simulink library "halin"  (R2021b)
settings: Solver=VariableStepAuto  StartTime=0.0  StopTime=10.0  RelTol=1e-3
undefined symbols (not defined in the file): KHAL_CAN1ABM1E2E_flg, KHAL_CAN1ESC1E2E_flg, KHAL_CAN1ESC5E2E_flg, KHAL_CAN1ESC7E2E_flg, KHAL_CAN1FCM2E2E_flg, KHAL_CAN1FCM3E2E_flg, KHAL_CAN1FCM4E2E_flg, KHAL_CAN3BMS1E2E_flg, KHAL_CAN3BMS6E2E_flg, KHAL_CAN3CCU1E2E_flg, KHAL_CAN3CCU2E2E_flg, KHAL_CAN3MCUF1E2E_flg, KHAL_CAN3MCUR1E2E_flg, KHAL_CAN3Shifter1E2E_flg, TRUE
libraries: simulink x420, FVT_lib x149, hcu_lib x49
(part 1 of 14)
settings Model: Creator=13168  LastModifiedBy=FVT23118
settings SolverCC: AlgebraicLoopSolver=TrustRegion
settings DataIOCC: SaveFormat=Array  SignalLoggingSaveFormat=ModelDataLogs  ReturnWorkspaceOutputs=off
settings OptimizationCC: BlockReduction=off  BooleanDataType=off
settings DebuggingCC: SaveWithParameterizedLinksMsg=none  UnderspecifiedInitializationDetection=Classic  MergeDetectMultiDrivingBlocksExec=none  SignalResolutionControl=TryResolveAllWithWarning  SFMachineParentedDataDiag=warning
settings HardwareCC: TargetUnknown=on
settings ModelReferenceCC: PropagateSignalLabelsOutOfModel=off
settings ConfigComp: CovMetricSettings=dw  CovSaveCumulativeToWorkspaceVar=on  CovSaveSingleToWorkspaceVar=on

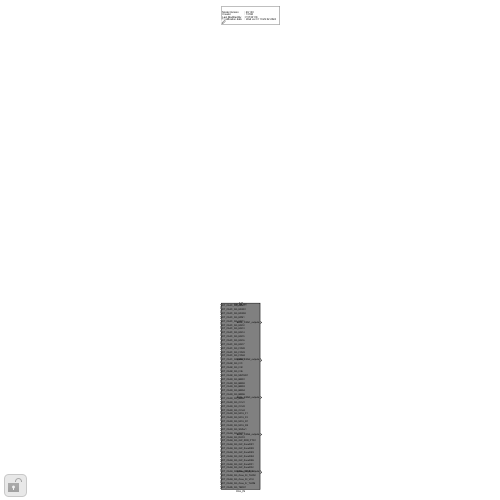
[thumbnail: Simulink's stored preview of the top-level diagram]
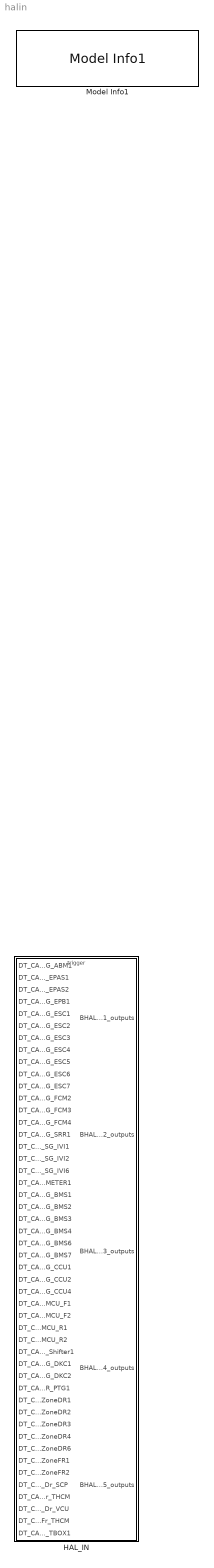
== system halin ==
  HAL_IN : Subsystem
      settings: RTWSystemCode=Nonreusable function  RTWFcnNameOpts=Use subsystem name  RTWFileNameOpts=Use subsystem name
  Model Info1 : hcu_lib/Model Info1  BlockCM=None  Frame=on  DisplayStringWithTags=|  HorizontalTextAlignment=Left  LeftAlignmentValue=0.02  SourceBlockDiagram=hcu_lib  TagMaxNumber=20
      | Model Version        : %<ModelVersion>
      | Creator                   : %<Creator>
      | Last Modified By    : %<LastModifiedBy>
      | Modification date    : %<LastModificationDate>
      settings: SourceProductName=HCU Relative Block Library

== system halin/HAL_IN ==
  DT_CAN1_SG_ABM1 : Inport
  DT_CAN1_SG_EPAS1 : Inport  Port=2
  DT_CAN1_SG_EPAS2 : Inport  Port=3
  DT_CAN1_SG_EPB1 : Inport  Port=4
  DT_CAN1_SG_ESC1 : Inport  Port=5
  DT_CAN1_SG_ESC2 : Inport  Port=6
  DT_CAN1_SG_ESC3 : Inport  Port=7
  DT_CAN1_SG_ESC4 : Inport  Port=8
  DT_CAN1_SG_ESC5 : Inport  Port=9
  DT_CAN1_SG_ESC6 : Inport  Port=10
  DT_CAN1_SG_ESC7 : Inport  Port=11
  DT_CAN1_SG_FCM2 : Inport  Port=12
  DT_CAN1_SG_FCM3 : Inport  Port=13
  DT_CAN1_SG_FCM4 : Inport  Port=14
  DT_CAN1_SG_SRR1 : Inport  Port=15
  DT_CAN2_SG_IVI1 : Inport  Port=16
  DT_CAN2_SG_IVI2 : Inport  Port=17
  DT_CAN2_SG_IVI6 : Inport  Port=18
  DT_CAN2_SG_METER1 : Inport  Port=19
  DT_CAN3_SG_BMS1 : Inport  Port=20
  DT_CAN3_SG_BMS2 : Inport  Port=21
  DT_CAN3_SG_BMS3 : Inport  Port=22
  DT_CAN3_SG_BMS4 : Inport  Port=23
  DT_CAN3_SG_BMS6 : Inport  Port=24
  DT_CAN3_SG_BMS7 : Inport  Port=25
  DT_CAN3_SG_CCU1 : Inport  Port=26
  DT_CAN3_SG_CCU2 : Inport  Port=27
  DT_CAN3_SG_CCU4 : Inport  Port=28
  DT_CAN3_SG_MCU_F1 : Inport  Port=29
  DT_CAN3_SG_MCU_F2 : Inport  Port=30
  DT_CAN3_SG_MCU_R1 : Inport  Port=31
  DT_CAN3_SG_MCU_R2 : Inport  Port=32
  DT_CAN3_SG_Shifter1 : Inport  Port=33
  DT_CAN4_SG_DKC1 : Inport  Port=34
  DT_CAN4_SG_DKC2 : Inport  Port=35
  DT_CAN4_SG_GW_ZDR_PTG1 : Inport  Port=36
  DT_CAN4_SG_GW_ZoneDR1 : Inport  Port=37
  DT_CAN4_SG_GW_ZoneDR2 : Inport  Port=38
  DT_CAN4_SG_GW_ZoneDR3 : Inport  Port=39
  DT_CAN4_SG_GW_ZoneDR4 : Inport  Port=40
  DT_CAN4_SG_GW_ZoneDR6 : Inport  Port=41
  DT_CAN4_SG_GW_ZoneFR1 : Inport  Port=42
  DT_CAN4_SG_GW_ZoneFR2 : Inport  Port=43
  DT_CAN4_SG_Zone_Dr_SCP : Inport  Port=44
  DT_CAN4_SG_Zone_Dr_THCM : Inport  Port=45
  DT_CAN4_SG_Zone_Dr_VCU : Inport  Port=46
  DT_CAN4_SG_Zone_Fr_THCM : Inport  Port=47
  DT_CAN5_SG_TBOX1 : Inport  Port=48
  trig_hal_in : TriggerPort  TriggerType=function-call  VariantControl=(inherit)
  CAN1 : Subsystem
  CAN2 : Subsystem
  CAN3 : Subsystem
  CAN4 : Subsystem
  CAN5 : Subsystem
  BHAL_CAN1_outputs : Outport  OutDataTypeStr=Bus: BHAL_CAN1_outputs
  BHAL_CAN2_outputs : Outport  Port=2  OutDataTypeStr=Bus: BHAL_CAN2_outputs
  BHAL_CAN3_outputs : Outport  Port=3  OutDataTypeStr=Bus: BHAL_CAN3_outputs
  BHAL_CAN4_outputs : Outport  Port=4  OutDataTypeStr=Bus: BHAL_CAN4_outputs
  BHAL_CAN5_outputs : Outport  Port=5  OutDataTypeStr=Bus: BHAL_CAN5_outputs
  wires:
  DT_CAN3_SG_CCU1/1 -> CAN3/7(DT_CAN3_SG_CCU1)
  DT_CAN3_SG_BMS3/1 -> CAN3/3(DT_CAN3_SG_BMS3)
  DT_CAN3_SG_BMS4/1 -> CAN3/4(DT_CAN3_SG_BMS4)
  DT_CAN3_SG_BMS2/1 -> CAN3/2(DT_CAN3_SG_BMS2)
  DT_CAN3_SG_MCU_R2/1 -> CAN3/13(DT_CAN3_SG_MCU_R2)
  DT_CAN3_SG_MCU_R1/1 -> CAN3/12(DT_CAN3_SG_MCU_R1)
  DT_CAN3_SG_BMS6/1 -> CAN3/5(DT_CAN3_SG_BMS6)
  DT_CAN3_SG_MCU_F1/1 -> CAN3/10(DT_CAN3_SG_MCU_F1)
  DT_CAN3_SG_MCU_F2/1 -> CAN3/11(DT_CAN3_SG_MCU_F2)
  DT_CAN3_SG_BMS1/1 -> CAN3/1(DT_CAN3_SG_BMS1)
  DT_CAN3_SG_CCU2/1 -> CAN3/8(DT_CAN3_SG_CCU2)
  DT_CAN4_SG_DKC2/1 -> CAN4/2(DT_CAN4_SG_DKC2)
  DT_CAN4_SG_DKC1/1 -> CAN4/1(DT_CAN4_SG_DKC1)
  DT_CAN4_SG_GW_ZDR_PTG1/1 -> CAN4/3(DT_CAN4_SG_GW_ZDR_PTG1)
  DT_CAN3_SG_CCU4/1 -> CAN3/9(DT_CAN3_SG_CCU4)
  DT_CAN4_SG_Zone_Dr_VCU/1 -> CAN4/13(DT_CAN4_SG_Zone_Dr_VCU)
  DT_CAN4_SG_Zone_Dr_SCP/1 -> CAN4/11(DT_CAN4_SG_Zone_Dr_SCP)
  DT_CAN4_SG_Zone_Dr_THCM/1 -> CAN4/12(DT_CAN4_SG_Zone_Dr_THCM)
  DT_CAN4_SG_GW_ZoneDR3/1 -> CAN4/6(DT_CAN4_SG_GW_ZoneDR3)
  CAN3/1(HAL_CAN3_outputs) -> BHAL_CAN3_outputs/1
  DT_CAN4_SG_GW_ZoneDR6/1 -> CAN4/8(DT_CAN4_SG_GW_ZoneDR6)
  CAN2/1(HAL_CAN2_outputs) -> BHAL_CAN2_outputs/1
  DT_CAN2_SG_METER1/1 -> CAN2/4(DT_CAN2_SG_METER1)
  DT_CAN4_SG_GW_ZoneFR1/1 -> CAN4/9(DT_CAN4_SG_GW_ZoneFR1)
  DT_CAN2_SG_IVI2/1 -> CAN2/2(DT_CAN2_SG_IVI2)
  DT_CAN2_SG_IVI1/1 -> CAN2/1(DT_CAN2_SG_IVI1)
  DT_CAN2_SG_IVI6/1 -> CAN2/3(DT_CAN2_SG_IVI6)
  DT_CAN1_SG_FCM3/1 -> CAN1/13(DT_CAN1_SG_FCM3)
  DT_CAN1_SG_FCM2/1 -> CAN1/12(DT_CAN1_SG_FCM2)
  DT_CAN1_SG_ESC7/1 -> CAN1/11(DT_CAN1_SG_ESC7)
  DT_CAN4_SG_GW_ZoneDR1/1 -> CAN4/4(DT_CAN4_SG_GW_ZoneDR1)
  DT_CAN1_SG_ESC6/1 -> CAN1/10(DT_CAN1_SG_ESC6)
  DT_CAN4_SG_GW_ZoneDR4/1 -> CAN4/7(DT_CAN4_SG_GW_ZoneDR4)
  DT_CAN3_SG_Shifter1/1 -> CAN3/14(DT_CAN3_SG_Shifter1)
  DT_CAN1_SG_ESC5/1 -> CAN1/9(DT_CAN1_SG_ESC5)
  DT_CAN4_SG_GW_ZoneFR2/1 -> CAN4/10(DT_CAN4_SG_GW_ZoneFR2)
  DT_CAN1_SG_ESC2/1 -> CAN1/6(DT_CAN1_SG_ESC2)
  DT_CAN1_SG_ESC3/1 -> CAN1/7(DT_CAN1_SG_ESC3)
  DT_CAN1_SG_ESC4/1 -> CAN1/8(DT_CAN1_SG_ESC4)
  DT_CAN1_SG_ESC1/1 -> CAN1/5(DT_CAN1_SG_ESC1)
  DT_CAN1_SG_EPAS2/1 -> CAN1/3(DT_CAN1_SG_EPAS2)
  DT_CAN4_SG_Zone_Fr_THCM/1 -> CAN4/14(DT_CAN4_SG_Zone_Fr_THCM)
  DT_CAN4_SG_GW_ZoneDR2/1 -> CAN4/5(DT_CAN4_SG_GW_ZoneDR2)
  DT_CAN1_SG_EPAS1/1 -> CAN1/2(DT_CAN1_SG_EPAS1)
  DT_CAN1_SG_EPB1/1 -> CAN1/4(DT_CAN1_SG_EPB1)
  CAN4/1(HAL_CAN4_outputs) -> BHAL_CAN4_outputs/1
  DT_CAN1_SG_SRR1/1 -> CAN1/15(DT_CAN1_SG_SRR1)
  DT_CAN1_SG_FCM4/1 -> CAN1/14(DT_CAN1_SG_FCM4)
  DT_CAN1_SG_ABM1/1 -> CAN1/1(DT_CAN1_SG_ABM1)
  DT_CAN5_SG_TBOX1/1 -> CAN5/1(DT_CAN5_SG_TBOX1)
  CAN1/1(HAL_CAN1_outputs) -> BHAL_CAN1_outputs/1
  CAN5/1(HAL_CAN5_outputs) -> BHAL_CAN5_outputs/1
  DT_CAN3_SG_BMS7/1 -> CAN3/6(DT_CAN3_SG_BMS7)

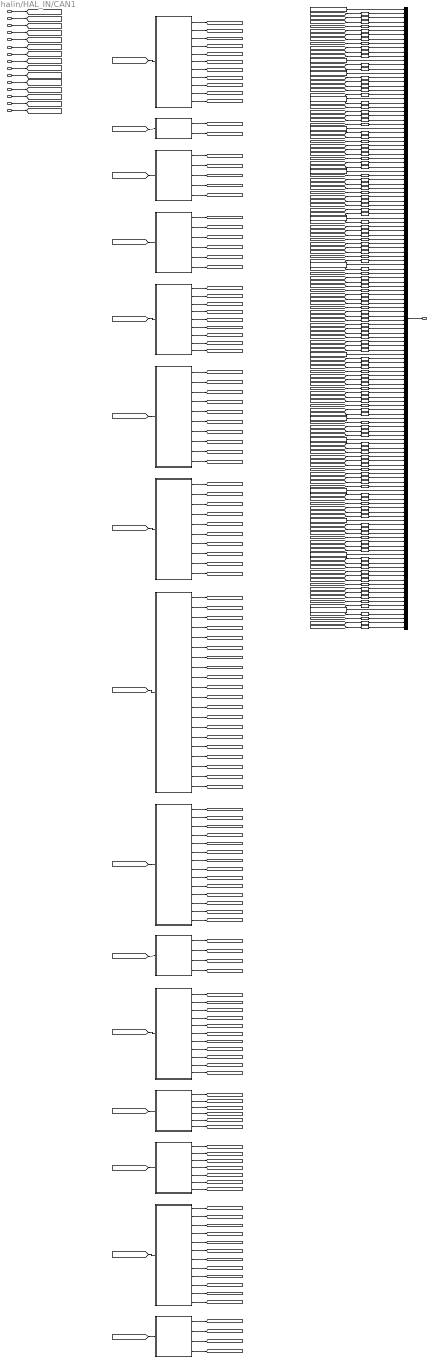
== system halin/HAL_IN/CAN1 ==
  DT_CAN1_SG_ABM1 : Inport
  DT_CAN1_SG_EPAS1 : Inport  Port=2
  DT_CAN1_SG_EPAS2 : Inport  Port=3
  DT_CAN1_SG_EPB1 : Inport  Port=4
  DT_CAN1_SG_ESC1 : Inport  Port=5
  DT_CAN1_SG_ESC2 : Inport  Port=6
  DT_CAN1_SG_ESC3 : Inport  Port=7
  DT_CAN1_SG_ESC4 : Inport  Port=8
  DT_CAN1_SG_ESC5 : Inport  Port=9
  DT_CAN1_SG_ESC6 : Inport  Port=10
  DT_CAN1_SG_ESC7 : Inport  Port=11
  DT_CAN1_SG_FCM2 : Inport  Port=12
  DT_CAN1_SG_FCM3 : Inport  Port=13
  DT_CAN1_SG_FCM4 : Inport  Port=14
  DT_CAN1_SG_SRR1 : Inport  Port=15
  ABM1 : Subsystem
  EPAS1 : Subsystem
  EPAS2 : Subsystem
  EPB1 : Subsystem
  ESC1 : Subsystem
  ESC2 : Subsystem
  ESC3 : Subsystem
  ESC4 : Subsystem
  ESC5 : Subsystem
  ESC6 : Subsystem
  ESC7 : Subsystem
  FCM2 : Subsystem
  FCM3 : Subsystem
  FCM4 : Subsystem
  SRR1 : Subsystem
  UnitConverter{,1..2,5,7..10,14,16..19,21..22,24..25,28,31,34,36,39,41,44,46,49,51,53..62,64..76,80,82,84,86..87,90..92,94,97,101..103,105,108..109,112,115..116,122..124} (72 alike) : DataTypeConversion  OutDataTypeStr=boolean
  UnitConverter{13,15,29..30,32,35,40,45,50,63,79,81,83,85,93,98,100,104,110..111} (20 alike) : DataTypeConversion  OutDataTypeStr=single
  UnitConverter{3..4,6,11..12,20,23,26..27,33,37..38,42..43,47..48,52,77..78,88..89,95..96,99,106..107,113..114,117..121,125..130} (39 alike) : DataTypeConversion  OutDataTypeStr=uint8
  VHAL_CANMsgInvalidABM1_flg : Subsystem  AncestorBlock=FVT_lib/hal/MsgTimeoutJudge_CAN_AUTOSAR
      mask help: MeasumentTrigerEvent
      mask Display: fprintf('MsgTimeoutJudge_CAN\nAUTOSAR');
  VHAL_CANMsgInvalidEPAS1_flg : Subsystem  AncestorBlock=FVT_lib/hal/MsgTimeoutJudge_CAN_AUTOSAR
      mask help: MeasumentTrigerEvent
      mask Display: fprintf('MsgTimeoutJudge_CAN\nAUTOSAR');
  VHAL_CANMsgInvalidEPAS2_flg : Subsystem  AncestorBlock=FVT_lib/hal/MsgTimeoutJudge_CAN_AUTOSAR
      mask help: MeasumentTrigerEvent
      mask Display: fprintf('MsgTimeoutJudge_CAN\nAUTOSAR');
  VHAL_CANMsgInvalidEPB1_flg : Subsystem  AncestorBlock=FVT_lib/hal/MsgTimeoutJudge_CAN_AUTOSAR
      mask help: MeasumentTrigerEvent
      mask Display: fprintf('MsgTimeoutJudge_CAN\nAUTOSAR');
  VHAL_CANMsgInvalidESC1_flg : Subsystem  AncestorBlock=FVT_lib/hal/MsgTimeoutJudge_CAN_AUTOSAR
      mask help: MeasumentTrigerEvent
      mask Display: fprintf('MsgTimeoutJudge_CAN\nAUTOSAR');
  VHAL_CANMsgInvalidESC2_flg : Subsystem  AncestorBlock=FVT_lib/hal/MsgTimeoutJudge_CAN_AUTOSAR
      mask help: MeasumentTrigerEvent
      mask Display: fprintf('MsgTimeoutJudge_CAN\nAUTOSAR');
  VHAL_CANMsgInvalidESC3_flg : Subsystem  AncestorBlock=FVT_lib/hal/MsgTimeoutJudge_CAN_AUTOSAR
      mask help: MeasumentTrigerEvent
      mask Display: fprintf('MsgTimeoutJudge_CAN\nAUTOSAR');
  VHAL_CANMsgInvalidESC4_flg : Subsystem  AncestorBlock=FVT_lib/hal/MsgTimeoutJudge_CAN_AUTOSAR
      mask help: MeasumentTrigerEvent
      mask Display: fprintf('MsgTimeoutJudge_CAN\nAUTOSAR');
  VHAL_CANMsgInvalidESC5_flg : Subsystem  AncestorBlock=FVT_lib/hal/MsgTimeoutJudge_CAN_AUTOSAR
      mask help: MeasumentTrigerEvent
      mask Display: fprintf('MsgTimeoutJudge_CAN\nAUTOSAR');
  VHAL_CANMsgInvalidESC6_flg : Subsystem  AncestorBlock=FVT_lib/hal/MsgTimeoutJudge_CAN_AUTOSAR
      mask help: MeasumentTrigerEvent
      mask Display: fprintf('MsgTimeoutJudge_CAN\nAUTOSAR');
  VHAL_CANMsgInvalidESC7_flg : Subsystem  AncestorBlock=FVT_lib/hal/MsgTimeoutJudge_CAN_AUTOSAR
      mask help: MeasumentTrigerEvent
      mask Display: fprintf('MsgTimeoutJudge_CAN\nAUTOSAR');
  VHAL_CANMsgInvalidFCM2_flg : Subsystem  AncestorBlock=FVT_lib/hal/MsgTimeoutJudge_CAN_AUTOSAR
      mask help: MeasumentTrigerEvent
      mask Display: fprintf('MsgTimeoutJudge_CAN\nAUTOSAR');
  VHAL_CANMsgInvalidFCM3_flg : Subsystem  AncestorBlock=FVT_lib/hal/MsgTimeoutJudge_CAN_AUTOSAR
      mask help: MeasumentTrigerEvent
      mask Display: fprintf('MsgTimeoutJudge_CAN\nAUTOSAR');
  VHAL_CANMsgInvalidFCM4_flg : Subsystem  AncestorBlock=FVT_lib/hal/MsgTimeoutJudge_CAN_AUTOSAR
      mask help: MeasumentTrigerEvent
      mask Display: fprintf('MsgTimeoutJudge_CAN\nAUTOSAR');
  VHAL_CANMsgInvalidSRR1_flg : Subsystem  AncestorBlock=FVT_lib/hal/MsgTimeoutJudge_CAN_AUTOSAR
      mask help: MeasumentTrigerEvent
      mask Display: fprintf('MsgTimeoutJudge_CAN\nAUTOSAR');
  bus_creator : BusCreator  Inputs=146
  HAL_CAN1_outputs : Outport
  wires:
  DT_CAN1_SG_ABM1/1 -> [DT_CAN1_SG_ABM1]
  DT_CAN1_SG_EPAS1/1 -> [DT_CAN1_SG_EPAS1]
  DT_CAN1_SG_EPAS2/1 -> [DT_CAN1_SG_EPAS2]
  DT_CAN1_SG_EPB1/1 -> [DT_CAN1_SG_EPB1]
  DT_CAN1_SG_ESC1/1 -> [DT_CAN1_SG_ESC1]
  DT_CAN1_SG_ESC2/1 -> [DT_CAN1_SG_ESC2]
  DT_CAN1_SG_ESC3/1 -> [DT_CAN1_SG_ESC3]
  DT_CAN1_SG_ESC4/1 -> [DT_CAN1_SG_ESC4]
  DT_CAN1_SG_ESC5/1 -> [DT_CAN1_SG_ESC5]
  DT_CAN1_SG_ESC6/1 -> [DT_CAN1_SG_ESC6]
  DT_CAN1_SG_ESC7/1 -> [DT_CAN1_SG_ESC7]
  DT_CAN1_SG_FCM2/1 -> [DT_CAN1_SG_FCM2]
  DT_CAN1_SG_FCM3/1 -> [DT_CAN1_SG_FCM3]
  DT_CAN1_SG_FCM4/1 -> [DT_CAN1_SG_FCM4]
  DT_CAN1_SG_SRR1/1 -> [DT_CAN1_SG_SRR1]
  [DT_CAN1_SG_ABM1] -> ABM1/1(DT_CAN1_SG_ABM1)
  [DT_CAN1_SG_EPAS1] -> EPAS1/1(DT_CAN1_SG_EPAS1)
  [DT_CAN1_SG_EPAS2] -> EPAS2/1(DT_CAN1_SG_EPAS2)
  [DT_CAN1_SG_EPB1] -> EPB1/1(DT_CAN1_SG_EPB1)
  [DT_CAN1_SG_ESC1] -> ESC1/1(DT_CAN1_SG_ESC1)
  [DT_CAN1_SG_ESC2] -> ESC2/1(DT_CAN1_SG_ESC2)
  [DT_CAN1_SG_ESC3] -> ESC3/1(DT_CAN1_SG_ESC3)
  [DT_CAN1_SG_ESC4] -> ESC4/1(DT_CAN1_SG_ESC4)
  [DT_CAN1_SG_ESC5] -> ESC5/1(DT_CAN1_SG_ESC5)
  [DT_CAN1_SG_ESC6] -> ESC6/1(DT_CAN1_SG_ESC6)
  [DT_CAN1_SG_ESC7] -> ESC7/1(DT_CAN1_SG_ESC7)
  [DT_CAN1_SG_FCM2] -> FCM2/1(DT_CAN1_SG_FCM2)
  [DT_CAN1_SG_FCM3] -> FCM3/1(DT_CAN1_SG_FCM3)
  [DT_CAN1_SG_FCM4] -> FCM4/1(DT_CAN1_SG_FCM4)
  [DT_CAN1_SG_SRR1] -> SRR1/1(DT_CAN1_SG_SRR1)
  bus_creator/1 -> HAL_CAN1_outputs/1
  VHAL_CANMsgInvalidABM1_flg/1(Out) -> bus_creator/1
  ABM1/1(VHAL_ABM1CSErr_flg) -> [VHAL_ABM1CSErr_flg]
  UnitConverter/1 -> bus_creator/2  "VHAL_ABM1CSErr_flg"
  [VHAL_ABM1CSErr_flg] -> UnitConverter/1
  ABM1/2(VHAL_ABM1RCErr_flg) -> [VHAL_ABM1RCErr_flg]
  UnitConverter1/1 -> bus_creator/3  "VHAL_ABM1RCErr_flg"
  [VHAL_ABM1RCErr_flg] -> UnitConverter1/1
  ABM1/3(VHAL_AirBagFailCmd_flg) -> [VHAL_AirBagFailCmd_flg]
  UnitConverter2/1 -> bus_creator/4  "VHAL_AirBagFailCmd_flg"
  [VHAL_AirBagFailCmd_flg] -> UnitConverter2/1
  ABM1/4(VHAL_ChecksumABM1_enum) -> [VHAL_ChecksumABM1_enum]
  UnitConverter3/1 -> bus_creator/5  "VHAL_ChecksumABM1_enum"
  [VHAL_ChecksumABM1_enum] -> UnitConverter3/1
  ABM1/5(VHAL_CrashOutputSts_enum) -> [VHAL_CrashOutputSts_enum]
  UnitConverter4/1 -> bus_creator/6  "VHAL_CrashOutputSts_enum"
  [VHAL_CrashOutputSts_enum] -> UnitConverter4/1
  ABM1/6(VHAL_DriverSeatBeltCmd_flg) -> [VHAL_DriverSeatBeltCmd_flg]
  UnitConverter5/1 -> bus_creator/7  "VHAL_DriverSeatBeltCmd_flg"
  [VHAL_DriverSeatBeltCmd_flg] -> UnitConverter5/1
  ABM1/7(VHAL_LifeCountABM1_enum) -> [VHAL_LifeCountABM1_enum]
  UnitConverter6/1 -> bus_creator/8  "VHAL_LifeCountABM1_enum"
  [VHAL_LifeCountABM1_enum] -> UnitConverter6/1
  ABM1/8(VHAL_PsngrSeatBeltCmd_flg) -> [VHAL_PsngrSeatBeltCmd_flg]
  UnitConverter7/1 -> bus_creator/9  "VHAL_PsngrSeatBeltCmd_flg"
  [VHAL_PsngrSeatBeltCmd_flg] -> UnitConverter7/1
  ABM1/9(VHAL_RCenterSeatBeltCmd_flg) -> [VHAL_RCenterSeatBeltCmd_flg]
  UnitConverter8/1 -> bus_creator/10  "VHAL_RCenterSeatBeltCmd_flg"
  [VHAL_RCenterSeatBeltCmd_flg] -> UnitConverter8/1
  ABM1/10(VHAL_RDriverSeatBeltCmd_flg) -> [VHAL_RDriverSeatBeltCmd_flg]
  UnitConverter9/1 -> bus_creator/11  "VHAL_RDriverSeatBeltCmd_flg"
  [VHAL_RDriverSeatBeltCmd_flg] -> UnitConverter9/1
  ABM1/11(VHAL_RPsngrSeatBeltCmd_flg) -> [VHAL_RPsngrSeatBeltCmd_flg]
  UnitConverter10/1 -> bus_creator/12  "VHAL_RPsngrSeatBeltCmd_flg"
  [VHAL_RPsngrSeatBeltCmd_flg] -> UnitConverter10/1
  VHAL_CANMsgInvalidEPAS1_flg/1(Out) -> bus_creator/13
  EPAS1/1(VHAL_DriIntend_enum) -> [VHAL_DriIntend_enum]
  UnitConverter11/1 -> bus_creator/14  "VHAL_DriIntend_enum"
  [VHAL_DriIntend_enum] -> UnitConverter11/1
  EPAS1/2(VHAL_EPSAOIControl_enum) -> [VHAL_EPSAOIControl_enum]
  UnitConverter12/1 -> bus_creator/15  "VHAL_EPSAOIControl_enum"
  [VHAL_EPSAOIControl_enum] -> UnitConverter12/1
  VHAL_CANMsgInvalidEPAS2_flg/1(Out) -> bus_creator/16
  EPAS2/1(VHAL_SASAngle_Deg) -> [VHAL_SASAngle_Deg]
  UnitConverter13/1 -> bus_creator/17  "VHAL_SASAngle_Deg"
  [VHAL_SASAngle_Deg] -> UnitConverter13/1
  EPAS2/2(VHAL_SASCAL_flg) -> [VHAL_SASCAL_flg]
  UnitConverter14/1 -> bus_creator/18  "VHAL_SASCAL_flg"
  [VHAL_SASCAL_flg] -> UnitConverter14/1
  EPAS2/3(VHAL_SASSpeed_degps) -> [VHAL_SASSpeed_degps]
  UnitConverter15/1 -> bus_creator/19  "VHAL_SASSpeed_degps"
  [VHAL_SASSpeed_degps] -> UnitConverter15/1
  EPAS2/4(VHAL_SASSpeedValid_flg) -> [VHAL_SASSpeedValid_flg]
  UnitConverter16/1 -> bus_creator/20  "VHAL_SASSpeedValid_flg"
  [VHAL_SASSpeedValid_flg] -> UnitConverter16/1
  EPAS2/5(VHAL_SASV_flg) -> [VHAL_SASV_flg]
  UnitConverter17/1 -> bus_creator/21  "VHAL_SASV_flg"
  [VHAL_SASV_flg] -> UnitConverter17/1
  VHAL_CANMsgInvalidEPB1_flg/1(Out) -> bus_creator/22
  EPB1/1(VHAL_DOASta_flg) -> [VHAL_DOASta_flg]
  UnitConverter18/1 -> bus_creator/23  "VHAL_DOASta_flg"
  [VHAL_DOASta_flg] -> UnitConverter18/1
  EPB1/2(VHAL_EPBCarWashMode_flg) -> [VHAL_EPBCarWashMode_flg]
  UnitConverter19/1 -> bus_creator/24  "VHAL_EPBCarWashMode_flg"
  [VHAL_EPBCarWashMode_flg] -> UnitConverter19/1
  EPB1/3(VHAL_EPBErrSta_enum) -> [VHAL_EPBErrSta_enum]
  UnitConverter20/1 -> bus_creator/25  "VHAL_EPBErrSta_enum"
  [VHAL_EPBErrSta_enum] -> UnitConverter20/1
  EPB1/4(VHAL_EPBExtApplyAvail_flg) -> [VHAL_EPBExtApplyAvail_flg]
  UnitConverter21/1 -> bus_creator/26  "VHAL_EPBExtApplyAvail_flg"
  [VHAL_EPBExtApplyAvail_flg] -> UnitConverter21/1
  EPB1/5(VHAL_EPBExtReleaseAvail_flg) -> [VHAL_EPBExtReleaseAvail_flg]
  UnitConverter22/1 -> bus_creator/27  "VHAL_EPBExtReleaseAvail_flg"
  [VHAL_EPBExtReleaseAvail_flg] -> UnitConverter22/1
  EPB1/6(VHAL_EPBSta_enum) -> [VHAL_EPBSta_enum]
  UnitConverter23/1 -> bus_creator/28  "VHAL_EPBSta_enum"
  [VHAL_EPBSta_enum] -> UnitConverter23/1
  VHAL_CANMsgInvalidESC1_flg/1(Out) -> bus_creator/29
  ESC1/1(VHAL_ESC1CSErr_flg) -> [VHAL_ESC1CSErr_flg]
  UnitConverter24/1 -> bus_creator/30  "VHAL_ESC1CSErr_flg"
  [VHAL_ESC1CSErr_flg] -> UnitConverter24/1
  ESC1/2(VHAL_ESC1RCErr_flg) -> [VHAL_ESC1RCErr_flg]
  UnitConverter25/1 -> bus_creator/31  "VHAL_ESC1RCErr_flg"
  [VHAL_ESC1RCErr_flg] -> UnitConverter25/1
  ESC1/3(VHAL_ESC1CS_enum) -> [VHAL_ESC1CS_enum]
  UnitConverter26/1 -> bus_creator/32  "VHAL_ESC1CS_enum"
  [VHAL_ESC1CS_enum] -> UnitConverter26/1
  ESC1/4(VHAL_ESC1RC_enum) -> [VHAL_ESC1RC_enum]
  UnitConverter27/1 -> bus_creator/33  "VHAL_ESC1RC_enum"
  [VHAL_ESC1RC_enum] -> UnitConverter27/1
  ESC1/5(VHAL_FrPTCSActive_flg) -> [VHAL_FrPTCSActive_flg]
  UnitConverter28/1 -> bus_creator/34  "VHAL_FrPTCSActive_flg"
  [VHAL_FrPTCSActive_flg] -> UnitConverter28/1
  ESC1/6(VHAL_FrntAxlTrqReqDrv_Nm) -> [VHAL_FrntAxlTrqReqDrv_Nm]
  UnitConverter29/1 -> bus_creator/35  "VHAL_FrntAxlTrqReqDrv_Nm"
  [VHAL_FrntAxlTrqReqDrv_Nm] -> UnitConverter29/1
  ESC1/7(VHAL_RearAxlTrqReqDrv_Nm) -> [VHAL_RearAxlTrqReqDrv_Nm]
  UnitConverter30/1 -> bus_creator/36  "VHAL_RearAxlTrqReqDrv_Nm"
  [VHAL_RearAxlTrqReqDrv_Nm] -> UnitConverter30/1
  ESC1/8(VHAL_RrPTCSActive_flg) -> [VHAL_RrPTCSActive_flg]
  UnitConverter31/1 -> bus_creator/37  "VHAL_RrPTCSActive_flg"
  [VHAL_RrPTCSActive_flg] -> UnitConverter31/1
  ESC1/9(VHAL_VehSpeed_kph) -> [VHAL_VehSpeed_kph]
  UnitConverter32/1 -> bus_creator/38  "VHAL_VehSpeed_kph"
  [VHAL_VehSpeed_kph] -> UnitConverter32/1
  VHAL_CANMsgInvalidESC2_flg/1(Out) -> bus_creator/39
  ESC2/1(VHAL_LFPulseCount_enum) -> [VHAL_LFPulseCount_enum]
  UnitConverter33/1 -> bus_creator/40  "VHAL_LFPulseCount_enum"
  [VHAL_LFPulseCount_enum] -> UnitConverter33/1
  ESC2/2(VHAL_LFPulseCountV_flg) -> [VHAL_LFPulseCountV_flg]
  UnitConverter34/1 -> bus_creator/41  "VHAL_LFPulseCountV_flg"
  [VHAL_LFPulseCountV_flg] -> UnitConverter34/1
  ESC2/3(VHAL_LFRawWhlSpeed_kph) -> [VHAL_LFRawWhlSpeed_kph]
  UnitConverter35/1 -> bus_creator/42  "VHAL_LFRawWhlSpeed_kph"
  [VHAL_LFRawWhlSpeed_kph] -> UnitConverter35/1
  ESC2/4(VHAL_LFRawWhlSpeedV_flg) -> [VHAL_LFRawWhlSpeedV_flg]
  UnitConverter36/1 -> bus_creator/43  "VHAL_LFRawWhlSpeedV_flg"
  [VHAL_LFRawWhlSpeedV_flg] -> UnitConverter36/1
  ESC2/5(VHAL_LFWhlRotDir_enum) -> [VHAL_LFWhlRotDir_enum]
  UnitConverter37/1 -> bus_creator/44  "VHAL_LFWhlRotDir_enum"
  [VHAL_LFWhlRotDir_enum] -> UnitConverter37/1
  ESC2/6(VHAL_RFPulseCount_enum) -> [VHAL_RFPulseCount_enum]
  UnitConverter38/1 -> bus_creator/45  "VHAL_RFPulseCount_enum"
  [VHAL_RFPulseCount_enum] -> UnitConverter38/1
  ESC2/7(VHAL_RFPulseCountV_flg) -> [VHAL_RFPulseCountV_flg]
  UnitConverter39/1 -> bus_creator/46  "VHAL_RFPulseCountV_flg"
  [VHAL_RFPulseCountV_flg] -> UnitConverter39/1
  ESC2/8(VHAL_RFRawWhlSpeed_kph) -> [VHAL_RFRawWhlSpeed_kph]
  UnitConverter40/1 -> bus_creator/47  "VHAL_RFRawWhlSpeed_kph"
  [VHAL_RFRawWhlSpeed_kph] -> UnitConverter40/1
  ESC2/9(VHAL_RFRawWhlSpeedV_flg) -> [VHAL_RFRawWhlSpeedV_flg]
  UnitConverter41/1 -> bus_creator/48  "VHAL_RFRawWhlSpeedV_flg"
  [VHAL_RFRawWhlSpeedV_flg] -> UnitConverter41/1
  ESC2/10(VHAL_RFWhlRotDir_enum) -> [VHAL_RFWhlRotDir_enum]
  UnitConverter42/1 -> bus_creator/49  "VHAL_RFWhlRotDir_enum"
  [VHAL_RFWhlRotDir_enum] -> UnitConverter42/1
  VHAL_CANMsgInvalidESC3_flg/1(Out) -> bus_creator/50
  ESC3/1(VHAL_LRPulseCount_enum) -> [VHAL_LRPulseCount_enum]
  UnitConverter43/1 -> bus_creator/51  "VHAL_LRPulseCount_enum"
  [VHAL_LRPulseCount_enum] -> UnitConverter43/1
  ESC3/2(VHAL_LRPulseCountV_flg) -> [VHAL_LRPulseCountV_flg]
  UnitConverter44/1 -> bus_creator/52  "VHAL_LRPulseCountV_flg"
  [VHAL_LRPulseCountV_flg] -> UnitConverter44/1
  ESC3/3(VHAL_LRRawWhlSpeed_kph) -> [VHAL_LRRawWhlSpeed_kph]
  UnitConverter45/1 -> bus_creator/53  "VHAL_LRRawWhlSpeed_kph"
  [VHAL_LRRawWhlSpeed_kph] -> UnitConverter45/1
  ESC3/4(VHAL_LRRawWhlSpeedV_flg) -> [VHAL_LRRawWhlSpeedV_flg]
  UnitConverter46/1 -> bus_creator/54  "VHAL_LRRawWhlSpeedV_flg"
  [VHAL_LRRawWhlSpeedV_flg] -> UnitConverter46/1
  ESC3/5(VHAL_LRWhlRotDir_enum) -> [VHAL_LRWhlRotDir_enum]
  UnitConverter47/1 -> bus_creator/55  "VHAL_LRWhlRotDir_enum"
  [VHAL_LRWhlRotDir_enum] -> UnitConverter47/1
  ESC3/6(VHAL_RRPulseCount_enum) -> [VHAL_RRPulseCount_enum]
  UnitConverter48/1 -> bus_creator/56  "VHAL_RRPulseCount_enum"
  [VHAL_RRPulseCount_enum] -> UnitConverter48/1
  ESC3/7(VHAL_RRPulseCountV_flg) -> [VHAL_RRPulseCountV_flg]
  UnitConverter49/1 -> bus_creator/57  "VHAL_RRPulseCountV_flg"
  [VHAL_RRPulseCountV_flg] -> UnitConverter49/1
  ESC3/8(VHAL_RRRawWhlSpeed_kph) -> [VHAL_RRRawWhlSpeed_kph]
  UnitConverter50/1 -> bus_creator/58  "VHAL_RRRawWhlSpeed_kph"
  [VHAL_RRRawWhlSpeed_kph] -> UnitConverter50/1
  ESC3/9(VHAL_RRRawWhlSpeedV_flg) -> [VHAL_RRRawWhlSpeedV_flg]
  UnitConverter51/1 -> bus_creator/59  "VHAL_RRRawWhlSpeedV_flg"
  [VHAL_RRRawWhlSpeedV_flg] -> UnitConverter51/1
  ESC3/10(VHAL_RRWhlRotDir_enum) -> [VHAL_RRWhlRotDir_enum]
  UnitConverter52/1 -> bus_creator/60  "VHAL_RRWhlRotDir_enum"
  [VHAL_RRWhlRotDir_enum] -> UnitConverter52/1
  VHAL_CANMsgInvalidESC4_flg/1(Out) -> bus_creator/61
  ESC4/1(VHAL_ABSActive_flg) -> [VHAL_ABSActive_flg]
  UnitConverter53/1 -> bus_creator/62  "VHAL_ABSActive_flg"
  [VHAL_ABSActive_flg] -> UnitConverter53/1
  ESC4/2(VHAL_ABSFailed_flg) -> [VHAL_ABSFailed_flg]
  UnitConverter54/1 -> bus_creator/63  "VHAL_ABSFailed_flg"
  [VHAL_ABSFailed_flg] -> UnitConverter54/1
  ESC4/3(VHAL_AVHActive_flg) -> [VHAL_AVHActive_flg]
  UnitConverter55/1 -> bus_creator/64  "VHAL_AVHActive_flg"
  [VHAL_AVHActive_flg] -> UnitConverter55/1
  ESC4/4(VHAL_AVHFailed_flg) -> [VHAL_AVHFailed_flg]
  UnitConverter56/1 -> bus_creator/65  "VHAL_AVHFailed_flg"
  [VHAL_AVHFailed_flg] -> UnitConverter56/1
  ESC4/5(VHAL_BTCSActive_flg) -> [VHAL_BTCSActive_flg]
  UnitConverter57/1 -> bus_creator/66  "VHAL_BTCSActive_flg"
  [VHAL_BTCSActive_flg] -> UnitConverter57/1
  ESC4/6(VHAL_EBDActive_flg) -> [VHAL_EBDActive_flg]
  UnitConverter58/1 -> bus_creator/67  "VHAL_EBDActive_flg"
  [VHAL_EBDActive_flg] -> UnitConverter58/1
  ESC4/7(VHAL_EBDFailed_flg) -> [VHAL_EBDFailed_flg]
  UnitConverter59/1 -> bus_creator/68  "VHAL_EBDFailed_flg"
  [VHAL_EBDFailed_flg] -> UnitConverter59/1
  ESC4/8(VHAL_ESCActive_flg) -> [VHAL_ESCActive_flg]
  UnitConverter60/1 -> bus_creator/69  "VHAL_ESCActive_flg"
  [VHAL_ESCActive_flg] -> UnitConverter60/1
  ESC4/9(VHAL_ESCFailed_flg) -> [VHAL_ESCFailed_flg]
  UnitConverter61/1 -> bus_creator/70  "VHAL_ESCFailed_flg"
  [VHAL_ESCFailed_flg] -> UnitConverter61/1
  ESC4/10(VHAL_ESSActive_flg) -> [VHAL_ESSActive_flg]
  UnitConverter62/1 -> bus_creator/71  "VHAL_ESSActive_flg"
  [VHAL_ESSActive_flg] -> UnitConverter62/1
  ESC4/11(VHAL_GRADE_Deg) -> [VHAL_GRADE_Deg]
  UnitConverter63/1 -> bus_creator/72  "VHAL_GRADE_Deg"
  [VHAL_GRADE_Deg] -> UnitConverter63/1
  ESC4/12(VHAL_HBBActive_flg) -> [VHAL_HBBActive_flg]
  UnitConverter64/1 -> bus_creator/73  "VHAL_HBBActive_flg"
  [VHAL_HBBActive_flg] -> UnitConverter64/1
  ESC4/13(VHAL_HBBFailed_flg) -> [VHAL_HBBFailed_flg]
  UnitConverter65/1 -> bus_creator/74  "VHAL_HBBFailed_flg"
  [VHAL_HBBFailed_flg] -> UnitConverter65/1
  ESC4/14(VHAL_HDDActive_flg) -> [VHAL_HDDActive_flg]
  UnitConverter66/1 -> bus_creator/75  "VHAL_HDDActive_flg"
  [VHAL_HDDActive_flg] -> UnitConverter66/1
  ESC4/15(VHAL_HDDFailed_flg) -> [VHAL_HDDFailed_flg]
  UnitConverter67/1 -> bus_creator/76  "VHAL_HDDFailed_flg"
  [VHAL_HDDFailed_flg] -> UnitConverter67/1
  ESC4/16(VHAL_HSAActive_flg) -> [VHAL_HSAActive_flg]
  UnitConverter68/1 -> bus_creator/77  "VHAL_HSAActive_flg"
  [VHAL_HSAActive_flg] -> UnitConverter68/1
  ESC4/17(VHAL_HSAFailed_flg) -> [VHAL_HSAFailed_flg]
  UnitConverter69/1 -> bus_creator/78  "VHAL_HSAFailed_flg"
  [VHAL_HSAFailed_flg] -> UnitConverter69/1
  ESC4/18(VHAL_PBAFailed_flg) -> [VHAL_PBAFailed_flg]
  UnitConverter70/1 -> bus_creator/79  "VHAL_PBAFailed_flg"
  [VHAL_PBAFailed_flg] -> UnitConverter70/1
  ESC4/19(VHAL_TCSActive_flg) -> [VHAL_TCSActive_flg]
  UnitConverter71/1 -> bus_creator/80  "VHAL_TCSActive_flg"
  [VHAL_TCSActive_flg] -> UnitConverter71/1
  ESC4/20(VHAL_TCSFailed_flg) -> [VHAL_TCSFailed_flg]
  UnitConverter72/1 -> bus_creator/81  "VHAL_TCSFailed_flg"
  [VHAL_TCSFailed_flg] -> UnitConverter72/1
  VHAL_CANMsgInvalidESC5_flg/1(Out) -> bus_creator/82
  ESC5/1(VHAL_ESC5CSErr_flg) -> [VHAL_ESC5CSErr_flg]
  UnitConverter73/1 -> bus_creator/83  "VHAL_ESC5CSErr_flg"
  [VHAL_ESC5CSErr_flg] -> UnitConverter73/1
  ESC5/2(VHAL_ESC5RCErr_flg) -> [VHAL_ESC5RCErr_flg]
  UnitConverter74/1 -> bus_creator/84  "VHAL_ESC5RCErr_flg"
  [VHAL_ESC5RCErr_flg] -> UnitConverter74/1
  ESC5/3(VHAL_BrkSwSta_flg) -> [VHAL_BrkSwSta_flg]
  UnitConverter75/1 -> bus_creator/85  "VHAL_BrkSwSta_flg"
  [VHAL_BrkSwSta_flg] -> UnitConverter75/1
  ESC5/4(VHAL_BrkSwV_flg) -> [VHAL_BrkSwV_flg]
  UnitConverter76/1 -> bus_creator/86  "VHAL_BrkSwV_flg"
  [VHAL_BrkSwV_flg] -> UnitConverter76/1
  ESC5/5(VHAL_ESC5CRC8_enum) -> [VHAL_ESC5CRC8_enum]
  UnitConverter77/1 -> bus_creator/87  "VHAL_ESC5CRC8_enum"
  [VHAL_ESC5CRC8_enum] -> UnitConverter77/1
  ESC5/6(VHAL_ESC5RC_enum) -> [VHAL_ESC5RC_enum]
  UnitConverter78/1 -> bus_creator/88  "VHAL_ESC5RC_enum"
  [VHAL_ESC5RC_enum] -> UnitConverter78/1
  ESC5/7(VHAL_LatAccel_Gps) -> [VHAL_LatAccel_Gps]
  UnitConverter79/1 -> bus_creator/89  "VHAL_LatAccel_Gps"
  [VHAL_LatAccel_Gps] -> UnitConverter79/1
  ESC5/8(VHAL_LatAccelV_flg) -> [VHAL_LatAccelV_flg]
  UnitConverter80/1 -> bus_creator/90  "VHAL_LatAccelV_flg"
  [VHAL_LatAccelV_flg] -> UnitConverter80/1
  ESC5/9(VHAL_LongAccel_Gps) -> [VHAL_LongAccel_Gps]
  UnitConverter81/1 -> bus_creator/91  "VHAL_LongAccel_Gps"
  [VHAL_LongAccel_Gps] -> UnitConverter81/1
  ESC5/10(VHAL_LongAccelV_flg) -> [VHAL_LongAccelV_flg]
  UnitConverter82/1 -> bus_creator/92  "VHAL_LongAccelV_flg"
  [VHAL_LongAccelV_flg] -> UnitConverter82/1
  ESC5/11(VHAL_MCPressure_bar) -> [VHAL_MCPressure_bar]
  UnitConverter83/1 -> bus_creator/93  "VHAL_MCPressure_bar"
  [VHAL_MCPressure_bar] -> UnitConverter83/1
  ESC5/12(VHAL_MCPressureV_flg) -> [VHAL_MCPressureV_flg]
  UnitConverter84/1 -> bus_creator/94  "VHAL_MCPressureV_flg"
  [VHAL_MCPressureV_flg] -> UnitConverter84/1
  ESC5/13(VHAL_YawRate_degps) -> [VHAL_YawRate_degps]
  UnitConverter85/1 -> bus_creator/95  "VHAL_YawRate_degps"
  [VHAL_YawRate_degps] -> UnitConverter85/1
  ESC5/14(VHAL_YawRateV_flg) -> [VHAL_YawRateV_flg]
  UnitConverter86/1 -> bus_creator/96  "VHAL_YawRateV_flg"
  [VHAL_YawRateV_flg] -> UnitConverter86/1
  VHAL_CANMsgInvalidESC6_flg/1(Out) -> bus_creator/97
  ESC6/1(VHAL_ActBrkLampSta_flg) -> [VHAL_ActBrkLampSta_flg]
  UnitConverter87/1 -> bus_creator/98  "VHAL_ActBrkLampSta_flg"
  [VHAL_ActBrkLampSta_flg] -> UnitConverter87/1
  ESC6/2(VHAL_ESCADASSta_enum) -> [VHAL_ESCADASSta_enum]
  UnitConverter88/1 -> bus_creator/99  "VHAL_ESCADASSta_enum"
  [VHAL_ESCADASSta_enum] -> UnitConverter88/1
  ESC6/3(VHAL_ESCAPSSta_enum) -> [VHAL_ESCAPSSta_enum]
  UnitConverter89/1 -> bus_creator/100  "VHAL_ESCAPSSta_enum"
  [VHAL_ESCAPSSta_enum] -> UnitConverter89/1
  ESC6/4(VHAL_ESCStandstill_flg) -> [VHAL_ESCStandstill_flg]
  UnitConverter90/1 -> bus_creator/101  "VHAL_ESCStandstill_flg"
  [VHAL_ESCStandstill_flg] -> UnitConverter90/1
  VHAL_CANMsgInvalidESC7_flg/1(Out) -> bus_creator/102
  ESC7/1(VHAL_ESC7CSErr_flg) -> [VHAL_ESC7CSErr_flg]
  UnitConverter91/1 -> bus_creator/103  "VHAL_ESC7CSErr_flg"
  [VHAL_ESC7CSErr_flg] -> UnitConverter91/1
  ESC7/2(VHAL_ESC7RCErr_flg) -> [VHAL_ESC7RCErr_flg]
  UnitConverter92/1 -> bus_creator/104  "VHAL_ESC7RCErr_flg"
  [VHAL_ESC7RCErr_flg] -> UnitConverter92/1
  ESC7/3(VHAL_BrkPedalPos_pct) -> [VHAL_BrkPedalPos_pct]
  UnitConverter93/1 -> bus_creator/105  "VHAL_BrkPedalPos_pct"
  [VHAL_BrkPedalPos_pct] -> UnitConverter93/1
  ESC7/4(VHAL_BrkPedalPosSta_flg) -> [VHAL_BrkPedalPosSta_flg]
  UnitConverter94/1 -> bus_creator/106  "VHAL_BrkPedalPosSta_flg"
  [VHAL_BrkPedalPosSta_flg] -> UnitConverter94/1
  ESC7/5(VHAL_ESC7CS_enum) -> [VHAL_ESC7CS_enum]
  UnitConverter95/1 -> bus_creator/107  "VHAL_ESC7CS_enum"
  [VHAL_ESC7CS_enum] -> UnitConverter95/1
  ESC7/6(VHAL_ESC7RC_enum) -> [VHAL_ESC7RC_enum]
  UnitConverter96/1 -> bus_creator/108  "VHAL_ESC7RC_enum"
  [VHAL_ESC7RC_enum] -> UnitConverter96/1
  ESC7/7(VHAL_FrRBCActive_flg) -> [VHAL_FrRBCActive_flg]
  UnitConverter97/1 -> bus_creator/109  "VHAL_FrRBCActive_flg"
  [VHAL_FrRBCActive_flg] -> UnitConverter97/1
  ESC7/8(VHAL_FrntAxlTrqReqBrk_Nm) -> [VHAL_FrntAxlTrqReqBrk_Nm]
  UnitConverter98/1 -> bus_creator/110  "VHAL_FrntAxlTrqReqBrk_Nm"
  [VHAL_FrntAxlTrqReqBrk_Nm] -> UnitConverter98/1
  ESC7/9(VHAL_RDCActive_enum) -> [VHAL_RDCActive_enum]
  UnitConverter99/1 -> bus_creator/111  "VHAL_RDCActive_enum"
  [VHAL_RDCActive_enum] -> UnitConverter99/1
  ESC7/10(VHAL_RearAxlTrqReqBrk_Nm) -> [VHAL_RearAxlTrqReqBrk_Nm]
  UnitConverter100/1 -> bus_creator/112  "VHAL_RearAxlTrqReqBrk_Nm"
  [VHAL_RearAxlTrqReqBrk_Nm] -> UnitConverter100/1
  ESC7/11(VHAL_RrRBCActive_flg) -> [VHAL_RrRBCActive_flg]
  UnitConverter101/1 -> bus_creator/113  "VHAL_RrRBCActive_flg"
  [VHAL_RrRBCActive_flg] -> UnitConverter101/1
  VHAL_CANMsgInvalidFCM2_flg/1(Out) -> bus_creator/114
  FCM2/1(VHAL_FCM2CSErr_flg) -> [VHAL_FCM2CSErr_flg]
  UnitConverter102/1 -> bus_creator/115  "VHAL_FCM2CSErr_flg"
  [VHAL_FCM2CSErr_flg] -> UnitConverter102/1
  FCM2/2(VHAL_FCM2RCErr_flg) -> [VHAL_FCM2RCErr_flg]
  UnitConverter103/1 -> bus_creator/116  "VHAL_FCM2RCErr_flg"
  [VHAL_FCM2RCErr_flg] -> UnitConverter103/1
  FCM2/3(VHAL_ACCRequiredAccel_mps2) -> [VHAL_ACCRequiredAccel_mps2]
  UnitConverter104/1 -> bus_creator/117  "VHAL_ACCRequiredAccel_mps2"
  [VHAL_ACCRequiredAccel_mps2] -> UnitConverter104/1
  FCM2/4(VHAL_ACCVehHoldReq_flg) -> [VHAL_ACCVehHoldReq_flg]
  UnitConverter105/1 -> bus_creator/118  "VHAL_ACCVehHoldReq_flg"
  [VHAL_ACCVehHoldReq_flg] -> UnitConverter105/1
  FCM2/5(VHAL_FCM2Checksum_enum) -> [VHAL_FCM2Checksum_enum]
  UnitConverter106/1 -> bus_creator/119  "VHAL_FCM2Checksum_enum"
  [VHAL_FCM2Checksum_enum] -> UnitConverter106/1
  FCM2/6(VHAL_FCM2LifeCount_enum) -> [VHAL_FCM2LifeCount_enum]
  UnitConverter107/1 -> bus_creator/120  "VHAL_FCM2LifeCount_enum"
  [VHAL_FCM2LifeCount_enum] -> UnitConverter107/1
  VHAL_CANMsgInvalidFCM3_flg/1(Out) -> bus_creator/121
  FCM3/1(VHAL_FCM3CSErr_flg) -> [VHAL_FCM3CSErr_flg]
  UnitConverter108/1 -> bus_creator/122  "VHAL_FCM3CSErr_flg"
  [VHAL_FCM3CSErr_flg] -> UnitConverter108/1
  FCM3/2(VHAL_FCM3RCErr_flg) -> [VHAL_FCM3RCErr_flg]
  UnitConverter109/1 -> bus_creator/123  "VHAL_FCM3RCErr_flg"
  [VHAL_FCM3RCErr_flg] -> UnitConverter109/1
  FCM3/3(VHAL_ACCObjDist_m) -> [VHAL_ACCObjDist_m]
  UnitConverter110/1 -> bus_creator/124  "VHAL_ACCObjDist_m"
  [VHAL_ACCObjDist_m] -> UnitConverter110/1
  FCM3/4(VHAL_ACCObjRelSpd_mps) -> [VHAL_ACCObjRelSpd_mps]
  UnitConverter111/1 -> bus_creator/125  "VHAL_ACCObjRelSpd_mps"
  [VHAL_ACCObjRelSpd_mps] -> UnitConverter111/1
  FCM3/5(VHAL_ADASForceIdle_flg) -> [VHAL_ADASForceIdle_flg]
  UnitConverter112/1 -> bus_creator/126  "VHAL_ADASForceIdle_flg"
  [VHAL_ADASForceIdle_flg] -> UnitConverter112/1
  FCM3/6(VHAL_FCM3Checksum_enum) -> [VHAL_FCM3Checksum_enum]
  UnitConverter113/1 -> bus_creator/127  "VHAL_FCM3Checksum_enum"
  [VHAL_FCM3Checksum_enum] -> UnitConverter113/1
  FCM3/7(VHAL_FCM3LifeCount_enum) -> [VHAL_FCM3LifeCount_enum]
  UnitConverter114/1 -> bus_creator/128  "VHAL_FCM3LifeCount_enum"
  [VHAL_FCM3LifeCount_enum] -> UnitConverter114/1
  VHAL_CANMsgInvalidFCM4_flg/1(Out) -> bus_creator/129
  FCM4/1(VHAL_FCM4CSErr_flg) -> [VHAL_FCM4CSErr_flg]
  UnitConverter115/1 -> bus_creator/130  "VHAL_FCM4CSErr_flg"
  [VHAL_FCM4CSErr_flg] -> UnitConverter115/1
  FCM4/2(VHAL_FCM4RCErr_flg) -> [VHAL_FCM4RCErr_flg]
  UnitConverter116/1 -> bus_creator/131  "VHAL_FCM4RCErr_flg"
  [VHAL_FCM4RCErr_flg] -> UnitConverter116/1
  FCM4/3(VHAL_ACCSetSpeed_enum) -> [VHAL_ACCSetSpeed_enum]
  UnitConverter117/1 -> bus_creator/132  "VHAL_ACCSetSpeed_enum"
  [VHAL_ACCSetSpeed_enum] -> UnitConverter117/1
  FCM4/4(VHAL_ACCSetSpeedDisp_enum) -> [VHAL_ACCSetSpeedDisp_enum]
  UnitConverter118/1 -> bus_creator/133  "VHAL_ACCSetSpeedDisp_enum"
  [VHAL_ACCSetSpeedDisp_enum] -> UnitConverter118/1
  FCM4/5(VHAL_ADASACCSta_enum) -> [VHAL_ADASACCSta_enum]
  UnitConverter119/1 -> bus_creator/134  "VHAL_ADASACCSta_enum"
  [VHAL_ADASACCSta_enum] -> UnitConverter119/1
  FCM4/6(VHAL_FCM4Checksum_enum) -> [VHAL_FCM4Checksum_enum]
  UnitConverter120/1 -> bus_creator/135  "VHAL_FCM4Checksum_enum"
  [VHAL_FCM4Checksum_enum] -> UnitConverter120/1
  FCM4/7(VHAL_ForceLowBeam_enum) -> [VHAL_ForceLowBeam_enum]
  UnitConverter121/1 -> bus_creator/136  "VHAL_ForceLowBeam_enum"
  [VHAL_ForceLowBeam_enum] -> UnitConverter121/1
  FCM4/8(VHAL_HazardWarningReq_flg) -> [VHAL_HazardWarningReq_flg]
  UnitConverter122/1 -> bus_creator/137  "VHAL_HazardWarningReq_flg"
  [VHAL_HazardWarningReq_flg] -> UnitConverter122/1
  FCM4/9(VHAL_LeftTurnLightReq_flg) -> [VHAL_LeftTurnLightReq_flg]
  UnitConverter123/1 -> bus_creator/138  "VHAL_LeftTurnLightReq_flg"
  [VHAL_LeftTurnLightReq_flg] -> UnitConverter123/1
  FCM4/10(VHAL_RightTurnLightReq_flg) -> [VHAL_RightTurnLightReq_flg]
  UnitConverter124/1 -> bus_creator/139  "VHAL_RightTurnLightReq_flg"
  [VHAL_RightTurnLightReq_flg] -> UnitConverter124/1
  FCM4/11(VHAL_TargetType_enum) -> [VHAL_TargetType_enum]
  UnitConverter125/1 -> bus_creator/140  "VHAL_TargetType_enum"
  [VHAL_TargetType_enum] -> UnitConverter125/1
  FCM4/12(VHAL_TimeGapLevel_enum) -> [VHAL_TimeGapLevel_enum]
  UnitConverter126/1 -> bus_creator/141  "VHAL_TimeGapLevel_enum"
  [VHAL_TimeGapLevel_enum] -> UnitConverter126/1
  VHAL_CANMsgInvalidSRR1_flg/1(Out) -> bus_creator/142
  SRR1/1(VHAL_SRRBSDWarnL_enum) -> [VHAL_SRRBSDWarnL_enum]
  UnitConverter127/1 -> bus_creator/143  "VHAL_SRRBSDWarnL_enum"
  [VHAL_SRRBSDWarnL_enum] -> UnitConverter127/1
  SRR1/2(VHAL_SRRBSDWarnR_enum) -> [VHAL_SRRBSDWarnR_enum]
  UnitConverter128/1 -> bus_creator/144  "VHAL_SRRBSDWarnR_enum"
  [VHAL_SRRBSDWarnR_enum] -> UnitConverter128/1
  SRR1/3(VHAL_SRRODAWarnL_enum) -> [VHAL_SRRODAWarnL_enum]
  UnitConverter129/1 -> bus_creator/145  "VHAL_SRRODAWarnL_enum"
  [VHAL_SRRODAWarnL_enum] -> UnitConverter129/1
  SRR1/4(VHAL_SRRODAWarnR_enum) -> [VHAL_SRRODAWarnR_enum]
  UnitConverter130/1 -> bus_creator/146  "VHAL_SRRODAWarnR_enum"
  [VHAL_SRRODAWarnR_enum] -> UnitConverter130/1
